simulink model "mech_jointlimit_prismatic"  (Simulink 7.1)
settings: Solver=ode23tb  StartTime=0.0  StopTime=10  RelTol=1e-3
libraries: mblibv1 x14, simulink x3
settings Model: Creator=arnav  LastModifiedBy=batserve
settings DebuggingCC: SaveWithParameterizedLinksMsg=none  SignalResolutionControl=TryResolveAllWithWarning  SolverPrmCheckMsg=none
settings GRTTargetCC: TargetFcnLib=ansi_tfl_tmw.mat
settings SimMechanicsCC: VisOnUpdateDiagram=on  VisDuringSimulation=on

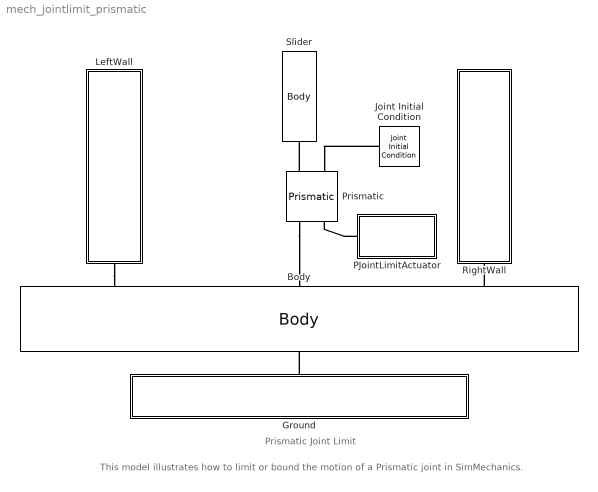
== system mech_jointlimit_prismatic ==
  note: Prismatic Joint Limit
  note: This model illustrates how to limit or bound the motion of a Prismatic joint in SimMechanics.
  Body : mblibv1/Bodies/Body  Orientation=down  DialogController=MECH.DynMechDlgSource  PhysicalDomain=mechanical  SubClassName=Unknown  LeftPortType=workingframe  RightPortType=workingframe  LConnTagsString=CS2|CS1|CS5  RConnTagsString=CG  DialogClass=MechanicalBodyBlock  Mass=1  MassUnits=kg  InertiaUnits=kg*m^2  Inertia=[0.05 0 0;0 0.75 0;0 0 0.705]  Shape=Cylinder  ShapeDims=[1 1]  ShapeUnits=m  ShapeUse=false  Density=1  DensityUnits=kg/m^3  DensityUse=false  GraphicsMode=1  BodyColor=[0.5 0.5 0.5]  GraphicsObj=[]  AttachedToCS=1  CG=Right$CG$[0 0 0]$Adjoining$Adjoining$m$[0 0 0]$Euler X-Y-Z$deg$WORLD$true  WorkingFrames=Left$CS2$[-1.5 0 0]$CS1$CS1$m$[0 0 0]$Euler X-Y-Z$deg$WORLD$true#Left$CS1$[0 0 0]$CG$CG$m$[0 0 0]$Euler X-Y-Z$deg$WORLD$true#Right$CS4$[-1.5 -0.5 0]$CS1$CS1$m$[0 0 0]$Euler X-Y-Z$deg$WORLD$false#Right$CS3$[1.5 -0.5 0]$CS1$CS1$m$[0 0 0]$Euler X-Y-Z$deg$WORLD$false#Left$CS5$[1.5 0 0]$CS1$CS1$m$[0 0 0]$Euler X-Y-Z$deg$WORLD$true  CGPos=[0 0 0]  CGRot=[0 0 0]  CS0Pos=[]  CS0Rot=[]  CS1Pos=[0 0 0]  CS1Rot=[0 0 0]  CS2Pos=[-1.5 0 0]  CS2Rot=[0 0 0]  CS3Pos=[1.5 -0.5 0]  CS3Rot=[0 0 0]  CS4Pos=[-1.5 -0.5 0]  CS4Rot=[0 0 0]  CS5Pos=[1.5 0 0]  CS5Rot=[0 0 0]  CS6Pos=[]  CS6Rot=[]  CS7Pos=[]  CS7Rot=[]  CS8Pos=[]  CS8Rot=[]  CS9Pos=[]  CS9Rot=[]  CS10Pos=[]  CS10Rot=[]  CS11Pos=[]  CS11Rot=[]  CS12Pos=[]  CS12Rot=[]  CS13Pos=[]  CS13Rot=[]  CS14Pos=[]  CS14Rot=[]  CS15Pos=[]  CS15Rot=[]  CS16Pos=[]  CS16Rot=[]  CS17Pos=[]  CS17Rot=[]  CS18Pos=[]  CS18Rot=[]  CS19Pos=[]  CS19Rot=[]  CS20Pos=[]  CS20Rot=[]
  Ground : Subsystem  Orientation=up
  Joint Initial Condition : mblibv1/Sensors &  Actuators/Joint Initial Condition  Orientation=left  DialogController=MECH.DynMechDlgSource  SystemSampleTime=-1  PhysicalDomain=mechanical  DialogClass=InitialConditionBlock  InitialConditions=P1$true$0$m$deg$1$m/s$deg/s#P2$false$0$m$deg$0$m/s$deg/s#P3$false$0$m$deg$0$m/s$deg/s#R1$false$0$m$deg$0$m/s$deg/s#R2$false$0$m$deg$0$m/s$deg/s#R3$false$0$m$deg$0$m/s$deg/s#S$false$0$m$deg$0$m/s$deg/s  P1PIC=0  P1VIC=1  P2PIC=0  P2VIC=0  P3PIC=0  P3VIC=0  R1PIC=0  R1VIC=0  R2PIC=0  R2VIC=0  R3PIC=0  R3VIC=0  SPIC=0  SVIC=0
  LeftWall : Subsystem  Orientation=up
  PJointLimitActuator : Subsystem  mask(Joint Limit){LHSLimit=1, RHSLimit=1, penDepth=0.0005, springC=2000, dampC=0.05}
      mask prompts: LHSLimit "LHS Joint Limit (m)"; RHSLimit "RHS Joint Limit (m)"; penDepth "Penetration Depth (m)"; springC "Spring Constant (N/m)"; dampC "Damping Constant (Ns/m)"
  Prismatic : mblibv1/Joints/Prismatic  Orientation=up  DialogController=MECH.DynMechDlgSource  PhysicalDomain=mechanical  SubClassName=Unknown  LeftPortType=blob  RightPortType=blob  LConnTagsString=__newl0|SA1  RConnTagsString=__newr0|SA1  NumSAPorts=2  CutJoint=off  MarkAsCut=off  Primitives=prismatic  PrimitiveProps=P1$World$[1 0 0]$prismatic  DialogClass=JointBlock  P1Axis=[1 0 0]
  RightWall : Subsystem  Orientation=up
  Slider : mblibv1/Bodies/Body  Orientation=down  DialogController=MECH.DynMechDlgSource  PhysicalDomain=mechanical  SubClassName=Unknown  LeftPortType=workingframe  RightPortType=workingframe  RConnTagsString=CS1  DialogClass=MechanicalBodyBlock  Mass=0.25  MassUnits=kg  InertiaUnits=kg*m^2  Inertia=[0.75 0 0;0 0.05 0;0 0 0.705]*0.035  Shape=Cylinder  ShapeDims=[1 1]  ShapeUnits=m  ShapeUse=false  Density=1  DensityUnits=kg/m^3  DensityUse=false  GraphicsMode=1  BodyColor=[0.5 0.5 0.5]  GraphicsObj=[]  AttachedToCS=1  CG=Right$CG$[0 0.625 0]$CS1$CS1$m$[0 0 0]$Euler X-Y-Z$deg$WORLD$false  WorkingFrames=Right$CS1$[0 0 0]$Adjoining$Adjoining$m$[0 0 0]$Euler X-Y-Z$deg$WORLD$true#Left$CS2$[0 1.25 0]$CS1$CS1$m$[0 0 0]$Euler X-Y-Z$deg$WORLD$false  CGPos=[0 0.625 0]  CGRot=[0 0 0]  CS0Pos=[]  CS0Rot=[]  CS1Pos=[0 0 0]  CS1Rot=[0 0 0]  CS2Pos=[0 1.25 0]  CS2Rot=[0 0 0]  CS3Pos=[]  CS3Rot=[]  CS4Pos=[]  CS4Rot=[]  CS5Pos=[]  CS5Rot=[]  CS6Pos=[]  CS6Rot=[]  CS7Pos=[]  CS7Rot=[]  CS8Pos=[]  CS8Rot=[]  CS9Pos=[]  CS9Rot=[]  CS10Pos=[]  CS10Rot=[]  CS11Pos=[]  CS11Rot=[]  CS12Pos=[]  CS12Rot=[]  CS13Pos=[]  CS13Rot=[]  CS14Pos=[]  CS14Rot=[]  CS15Pos=[]  CS15Rot=[]  CS16Pos=[]  CS16Rot=[]  CS17Pos=[]  CS17Rot=[]  CS18Pos=[]  CS18Rot=[]  CS19Pos=[]  CS19Rot=[]  CS20Pos=[]  CS20Rot=[]
  connections:
  Prismatic/RConn1 -- Slider/RConn1
  Ground/RConn1 -- Body/RConn1
  Body/LConn3 -- RightWall/LConn1
  LeftWall/LConn1 -- Body/LConn1
  PJointLimitActuator/LConn1 -- Prismatic/LConn2
  Joint Initial Condition/RConn1 -- Prismatic/RConn2
  Prismatic/LConn1 -- Body/LConn2

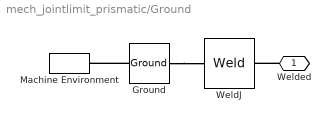
== system mech_jointlimit_prismatic/Ground ==
  Ground : mblibv1/Bodies/Ground  DialogController=MECH.DynMechDlgSource  SystemSampleTime=-1  LeftPortType=env  RightPortType=workingframe  PhysicalDomain=Mechanical  DialogClass=GroundBlock  CoordPosition=[0 0 0]  CoordPositionUnits=m  StateVectorMgrId=-1  MachineId=[0 0]  ShowEnvPort=on
  Machine Environment : mblibv1/Bodies/Machine Environment  Tag=Factory ground  DialogController=MECH.DialogSource  SystemSampleTime=-1  PortType=env  PhysicalDomain=Mechanical  DialogTemplateClass=MECH.MachineEnvironment  SyncWhenCopied=off  Gravity=[0 -9.81 0]  GravityUnits=m/s^2  GravityAsSignal=off  Dimensionality=Auto-detect  AnalysisType=Forward dynamics  LinearAssemblyTolerance=1e-3  LinearAssemblyToleranceUnits=m  AngularAssemblyTolerance=1e-3  AngularAssemblyToleranceUnits=rad  ConstraintSolverType=Stabilizing  ConstraintRelTolerance=1e-4  ConstraintAbsTolerance=1e-4  UseRobustSingularityHandling=off  RedundancyAnalysisToleranceType=Automatically select tolerance  RedundancyAnalysisTolerance=1e-14  StatePerturbationType=Fixed  PerturbationSize=1e-5  VisualizeMachine=on
  WeldJ : mblibv1/Joints/Weld  DialogController=MECH.DynMechDlgSource  PhysicalDomain=mechanical  SubClassName=Unknown  LeftPortType=blob  RightPortType=blob  LConnTagsString=__newl0  RConnTagsString=__newr0  NumSAPorts=0  CutJoint=off  MarkAsCut=off  Primitives=weld  PrimitiveProps=W$WORLD$[0 0 0]$weld  DialogClass=JointBlock  WAxis=[0 0 0]
  Welded : PMIOPort  Orientation=left  Port=1  Side=Right
  connections:
  Ground/LConn1 -- Machine Environment/RConn1
  Ground/RConn1 -- WeldJ/LConn1
  Welded/RConn1 -- WeldJ/RConn1

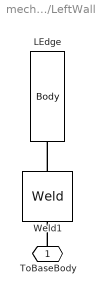
== system mech_jointlimit_prismatic/LeftWall ==
  LEdge : mblibv1/Bodies/Body  Orientation=down  DialogController=MECH.DynMechDlgSource  PhysicalDomain=mechanical  SubClassName=Unknown  LeftPortType=workingframe  RightPortType=workingframe  RConnTagsString=CS1  DialogClass=MechanicalBodyBlock  Mass=0.2  MassUnits=kg  InertiaUnits=kg*m^2  Inertia=[0.75 0 0;0 0.05 0;0 0 0.705]*0.02  Shape=Cylinder  ShapeDims=[1 1]  ShapeUnits=m  ShapeUse=false  Density=1  DensityUnits=kg/m^3  DensityUse=false  GraphicsMode=1  BodyColor=[0.5 0.5 0.5]  GraphicsObj=[]  AttachedToCS=1  CG=Right$CG$[0.4 0.5 0]$CS1$CS1$m$[0 0 0]$Euler X-Y-Z$deg$WORLD$false  WorkingFrames=Right$CS1$[0 0 0]$Adjoining$Adjoining$m$[0 0 0]$Euler X-Y-Z$deg$WORLD$true#Left$CS2$[0 1 0]$CS1$CS1$m$[0 0 0]$Euler X-Y-Z$deg$WORLD$false#Right$CS4$[0.5 1 0]$CS1$CS1$m$[0 0 0]$Euler X-Y-Z$deg$WORLD$false#Right$CS3$[0.5 0 0]$CS1$CS1$m$[0 0 0]$Euler X-Y-Z$deg$WORLD$false  CGPos=[0.4 0.5 0]  CGRot=[0 0 0]  CS0Pos=[]  CS0Rot=[]  CS1Pos=[0 0 0]  CS1Rot=[0 0 0]  CS2Pos=[0 1 0]  CS2Rot=[0 0 0]  CS3Pos=[0.5 0 0]  CS3Rot=[0 0 0]  CS4Pos=[0.5 1 0]  CS4Rot=[0 0 0]  CS5Pos=[]  CS5Rot=[]  CS6Pos=[]  CS6Rot=[]  CS7Pos=[]  CS7Rot=[]  CS8Pos=[]  CS8Rot=[]  CS9Pos=[]  CS9Rot=[]  CS10Pos=[]  CS10Rot=[]  CS11Pos=[]  CS11Rot=[]  CS12Pos=[]  CS12Rot=[]  CS13Pos=[]  CS13Rot=[]  CS14Pos=[]  CS14Rot=[]  CS15Pos=[]  CS15Rot=[]  CS16Pos=[]  CS16Rot=[]  CS17Pos=[]  CS17Rot=[]  CS18Pos=[]  CS18Rot=[]  CS19Pos=[]  CS19Rot=[]  CS20Pos=[]  CS20Rot=[]
  Weld1 : mblibv1/Joints/Weld  Orientation=up  DialogController=MECH.DynMechDlgSource  PhysicalDomain=mechanical  SubClassName=Unknown  LeftPortType=blob  RightPortType=blob  LConnTagsString=__newl0  RConnTagsString=__newr0  NumSAPorts=0  CutJoint=off  MarkAsCut=off  Primitives=weld  PrimitiveProps=W$WORLD$[0 0 0]$weld  DialogClass=JointBlock  WAxis=[0 0 0]
  ToBaseBody : PMIOPort  Orientation=up  Port=1  Side=Left
  connections:
  Weld1/RConn1 -- LEdge/RConn1
  ToBaseBody/RConn1 -- Weld1/LConn1

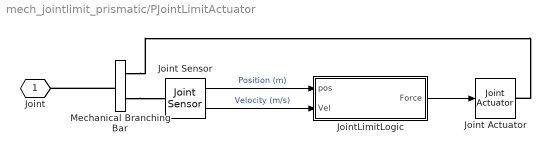
== system mech_jointlimit_prismatic/PJointLimitActuator ==
  Joint Actuator : mblibv1/Sensors &  Actuators/Joint Actuator  DialogController=MECH.DynMechDlgSource  SystemSampleTime=-1  PhysicalDomain=Mechanical  PortType=blob  ActuationStyle=Force  AngleUnits=deg  ArcVelocityUnits=deg/s  ArcAccelerationUnits=deg/s^2  CoordPositionUnits=m  VelocityUnits=m/s  AccelerationUnits=m/s^2  ForceUnits=N  TorqueUnits=N*m  ActiveIO=on  Width=1  DialogClass=MechanicalActuatorBlock  Primitive=P1  ReferenceFrame=Absolute (INERTIAL)
  Joint Sensor : mblibv1/Sensors &  Actuators/Joint Sensor  DialogController=MECH.DynMechDlgSource  SystemSampleTime=-1  PhysicalDomain=Mechanical  PortType=blob  Muxed=off  Pose=off  Angle=on  AngleUnits=rad  ArcVelocity=on  ArcVelocityUnits=rad/s  ArcAcceleration=off  ArcAccelerationUnits=deg/s^2  CoordPosition=on  CoordPositionUnits=m  Velocity=on  VelocityUnits=m/s  Acceleration=off  AccelerationUnits=m/s^2  Quaternion=off  QuaternionDT=off  QuaternionDDT=off  QuaternionUnits=off  OutputVector=[ 1 1 ]  ActiveIO=on  Width=2  DialogClass=MechanicalSensorBlock  Primitive=P1  Force=off  ForceUnits=N  Torque=off  TorqueUnits=N*m  ReferenceFrame=Absolute (INERTIAL)  ReactionSensedSide=Base  ReactionReferenceFrame=Absolute (World)  ReactionForce=off  ReactionForceUnits=N  ReactionMoment=off  ReactionMomentUnits=N*m
  JointLimitLogic : Subsystem
  Mechanical Branching Bar : mblibv1/Utilities/Mechanical Branching Bar  DialogController=MECH.DynMechDlgSource  PhysicalDomain=mechanical  SubClassName=Unknown  LeftPortType=blob  RightPortType=blob  LConnTagsString=_newl0  RConnTagsString=SA0|SA1  DialogClass=MechanicalBranchingBarBlock  NumSAPorts=2
  Joint : PMIOPort  Tag=PMCPort  Port=1  Side=Left
  wires:
  Joint Sensor/1 -> JointLimitLogic/1(pos)  "Position (m)"
  Joint Sensor/2 -> JointLimitLogic/2(Vel)  "Velocity (m/s)"
  JointLimitLogic/1(Force) -> Joint Actuator/1
  connections:
  Mechanical Branching Bar/LConn1 -- Joint/RConn1
  Mechanical Branching Bar/RConn2 -- Joint Sensor/LConn1
  Mechanical Branching Bar/RConn1 -- Joint Actuator/RConn1

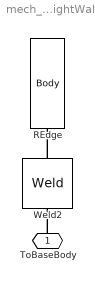
== system mech_jointlimit_prismatic/RightWall ==
  REdge : mblibv1/Bodies/Body  Orientation=down  DialogController=MECH.DynMechDlgSource  PhysicalDomain=mechanical  SubClassName=Unknown  LeftPortType=workingframe  RightPortType=workingframe  RConnTagsString=CS1  DialogClass=MechanicalBodyBlock  Mass=0.2  MassUnits=kg  InertiaUnits=kg*m^2  Inertia=[0.75 0 0;0 0.05 0;0 0 0.705]*0.02  Shape=Cylinder  ShapeDims=[1 1]  ShapeUnits=m  ShapeUse=false  Density=1  DensityUnits=kg/m^3  DensityUse=false  GraphicsMode=1  BodyColor=[0.5 0.5 0.5]  GraphicsObj=[]  AttachedToCS=1  CG=Right$CG$[-0.4 0.5 0]$CS1$CS1$m$[0 0 0]$Euler X-Y-Z$deg$WORLD$false  WorkingFrames=Right$CS1$[0 0 0]$Adjoining$Adjoining$m$[0 0 0]$Euler X-Y-Z$deg$WORLD$true#Left$CS2$[0 1 0]$CS1$CS1$m$[0 0 0]$Euler X-Y-Z$deg$WORLD$false#Right$CS4$[-0.5 1 0]$CS1$CS1$m$[0 0 0]$Euler X-Y-Z$deg$WORLD$false#Right$CS3$[-0.5 0 0]$CS1$CS1$m$[0 0 0]$Euler X-Y-Z$deg$WORLD$false  CGPos=[-0.4 0.5 0]  CGRot=[0 0 0]  CS0Pos=[]  CS0Rot=[]  CS1Pos=[0 0 0]  CS1Rot=[0 0 0]  CS2Pos=[0 1 0]  CS2Rot=[0 0 0]  CS3Pos=[-0.5 0 0]  CS3Rot=[0 0 0]  CS4Pos=[-0.5 1 0]  CS4Rot=[0 0 0]  CS5Pos=[]  CS5Rot=[]  CS6Pos=[]  CS6Rot=[]  CS7Pos=[]  CS7Rot=[]  CS8Pos=[]  CS8Rot=[]  CS9Pos=[]  CS9Rot=[]  CS10Pos=[]  CS10Rot=[]  CS11Pos=[]  CS11Rot=[]  CS12Pos=[]  CS12Rot=[]  CS13Pos=[]  CS13Rot=[]  CS14Pos=[]  CS14Rot=[]  CS15Pos=[]  CS15Rot=[]  CS16Pos=[]  CS16Rot=[]  CS17Pos=[]  CS17Rot=[]  CS18Pos=[]  CS18Rot=[]  CS19Pos=[]  CS19Rot=[]  CS20Pos=[]  CS20Rot=[]
  Weld2 : mblibv1/Joints/Weld  Orientation=up  DialogController=MECH.DynMechDlgSource  PhysicalDomain=mechanical  SubClassName=Unknown  LeftPortType=blob  RightPortType=blob  LConnTagsString=__newl0  RConnTagsString=__newr0  NumSAPorts=0  CutJoint=off  MarkAsCut=off  Primitives=weld  PrimitiveProps=W$WORLD$[0 0 0]$weld  DialogClass=JointBlock  WAxis=[0 0 0]
  ToBaseBody : PMIOPort  Orientation=up  Port=1  Side=Left
  connections:
  Weld2/RConn1 -- REdge/RConn1
  ToBaseBody/RConn1 -- Weld2/LConn1

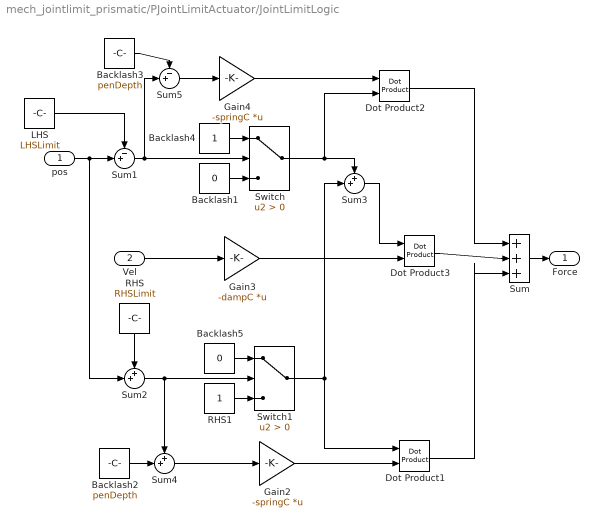
== system mech_jointlimit_prismatic/PJointLimitActuator/JointLimitLogic ==
  pos : Inport  OutDataType=sfix(16)  OutScaling=2^0
  Vel : Inport  Port=2  OutDataType=sfix(16)  OutScaling=2^0
  Backlash1 : Constant  Value=0  OutDataType=sfix(16)  OutScaling=2^0
  Backlash2 : Constant  Value=penDepth  OutDataType=sfix(16)  OutScaling=2^0
  Backlash3 : Constant  Value=penDepth  OutDataType=sfix(16)  OutScaling=2^0
  Backlash4 : Constant  OutDataType=sfix(16)  OutScaling=2^0
  Backlash5 : Constant  Value=0  OutDataType=sfix(16)  OutScaling=2^0
  Dot Product1 : simulink/Math Operations/Dot Product  InputSameDT=on  OutDataType=sfix(16)  OutScaling=2^-10  DoSatur=off
  Dot Product2 : simulink/Math Operations/Dot Product  InputSameDT=on  OutDataType=sfix(16)  OutScaling=2^-10  DoSatur=off
  Dot Product3 : simulink/Math Operations/Dot Product  InputSameDT=on  OutDataType=sfix(16)  OutScaling=2^-10  DoSatur=off
  Gain2 : Gain  Gain=-springC  Multiplication=Matrix(K*u)  ParameterDataType=sfix(16)  ParameterScaling=2^0  OutDataType=sfix(16)  OutScaling=2^0  SaturateOnIntegerOverflow=on  OutDataTypeStr=Inherit: Same as input  ParamDataTypeStr=Inherit: Same as input
  Gain3 : Gain  Gain=-dampC  Multiplication=Matrix(K*u)  ParameterDataType=sfix(16)  ParameterScaling=2^0  OutDataType=sfix(16)  OutScaling=2^0  SaturateOnIntegerOverflow=on  OutDataTypeStr=Inherit: Same as input  ParamDataTypeStr=Inherit: Same as input
  Gain4 : Gain  Gain=-springC  Multiplication=Matrix(K*u)  ParameterDataType=sfix(16)  ParameterScaling=2^0  OutDataType=sfix(16)  OutScaling=2^0  SaturateOnIntegerOverflow=on  OutDataTypeStr=Inherit: Same as input  ParamDataTypeStr=Inherit: Same as input
  LHS : Constant  Value=LHSLimit  OutDataType=sfix(16)  OutScaling=2^0
  RHS : Constant  Orientation=down  Value=RHSLimit  OutDataType=sfix(16)  OutScaling=2^0
  RHS1 : Constant  OutDataType=sfix(16)  OutScaling=2^0
  Sum : Sum  Inputs=+++|  OutDataType=sfix(16)  OutScaling=2^0  SaturateOnIntegerOverflow=on
  Sum1 : Sum  Inputs=-+|  OutDataType=sfix(16)  OutScaling=2^0  SaturateOnIntegerOverflow=on
  Sum2 : Sum  Inputs=++|  OutDataType=sfix(16)  OutScaling=2^0  SaturateOnIntegerOverflow=on
  Sum3 : Sum  Inputs=++|  OutDataType=sfix(16)  OutScaling=2^0  SaturateOnIntegerOverflow=on
  Sum4 : Sum  Inputs=++|  OutDataType=sfix(16)  OutScaling=2^0  SaturateOnIntegerOverflow=on
  Sum5 : Sum  Inputs=-+|  OutDataType=sfix(16)  OutScaling=2^0  SaturateOnIntegerOverflow=on
  Switch : Switch  Criteria=u2 > Threshold
  Switch1 : Switch  Criteria=u2 > Threshold
  Force : Outport  OutDataType=sfix(16)  OutScaling=2^0
  wires:
  pos/1 -> Sum1/2, Sum2/2
  LHS/1 -> Sum1/1
  Sum1/1 -> Switch/2, Sum5/2
  Backlash1/1 -> Switch/3
  RHS/1 -> Sum2/1
  Sum2/1 -> Switch1/2, Sum4/1
  RHS1/1 -> Switch1/3
  Backlash4/1 -> Switch/1
  Switch/1 -> Dot Product2/2, Sum3/1
  Switch1/1 -> Dot Product1/1, Sum3/2
  Backlash5/1 -> Switch1/1
  Vel/1 -> Gain3/1
  Backlash2/1 -> Sum4/2
  Sum4/1 -> Gain2/1
  Gain2/1 -> Dot Product1/2
  Backlash3/1 -> Sum5/1
  Sum5/1 -> Gain4/1
  Gain4/1 -> Dot Product2/1
  Dot Product1/1 -> Sum/3
  Sum/1 -> Force/1
  Dot Product2/1 -> Sum/1
  Gain3/1 -> Dot Product3/2
  Sum3/1 -> Dot Product3/1
  Dot Product3/1 -> Sum/2
